simulink model "LoadFlow116BusNetwork_original"  (R2024a)
settings: Solver=FixedStepDiscrete  StartTime=0.0  StopTime=4.5  FixedStep=75e-6  RelTol=1e-3  EnableMultiTasking=on
undefined symbols (not defined in the file or in its folder): D1, D11, Delta
libraries: spsSeriesRLCBranchLib x164, spsLoadFlowBusLib x116, spsDistributedParametersLineLib x79, spsThreePhaseSeriesRLCLoadLib x60, spsThreePhaseTransformerTwoWindingsLib x52, spsThreePhaseParallelRLCLoadLib x44, spsThreePhaseVIMeasurementLib x44, spsSynchronousMachinepuStandardLib x28, spsExcitationSystemLib x28, spsHydraulicTurbineandGovernorLib x28, spsGenericPowerSystemStabilizerLib x28, spsMultiBandPowerSystemStabilizerLib x28
(part 9 of 15)

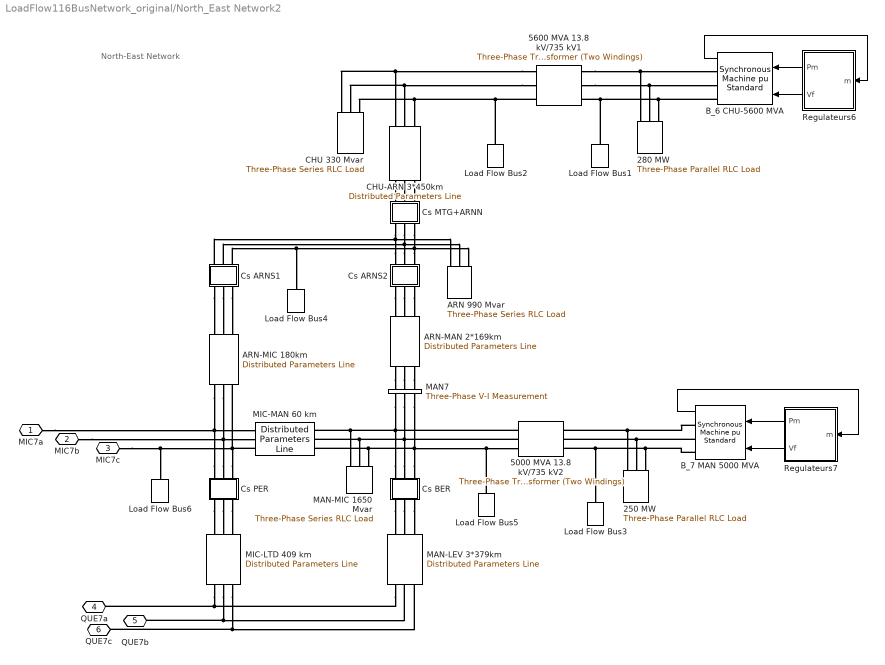
== system LoadFlow116BusNetwork_original/North_East Network2 ==
  note: North-East Network
  250 MW : spsThreePhaseParallelRLCLoadLib/Three-Phase Parallel RLC Load  LConnTagsString=A|B|C  Configuration=Y (grounded)  NominalVoltage=(13800)*1  Vabc=[1e3 1e3 1e3]  Vabcp=[1e3 1e3 1e3]  NominalFrequency=60  UnbalancedPower=off  ActivePower=250000000  InductivePower=0  CapacitivePower=0  Pabc=[10e3 9e3 11e3]  QLabc=[100 90 110]  QCabc=[100 90 110]  Pabcp=[10e3 9e3 11e3]  QLabcp=[100 90 110]  QCabcp=[100 90 110]  Measurements=None  LoadType=constant PQ
  280 MW : spsThreePhaseParallelRLCLoadLib/Three-Phase Parallel RLC Load  LConnTagsString=A|B|C  Configuration=Y (grounded)  NominalVoltage=(13800)*1  Vabc=[1e3 1e3 1e3]  Vabcp=[1e3 1e3 1e3]  NominalFrequency=60  UnbalancedPower=off  ActivePower=280000000  InductivePower=0  CapacitivePower=0  Pabc=[10e3 9e3 11e3]  QLabc=[100 90 110]  QCabc=[100 90 110]  Pabcp=[10e3 9e3 11e3]  QLabcp=[100 90 110]  QCabcp=[100 90 110]  Measurements=None  LoadType=constant PQ
  5000 MVA 13.8 kV/735 kV2 : spsThreePhaseTransformerTwoWindingsLib/Three-Phase Transformer (Two Windings)  Winding1Connection=Delta (D1)  Winding2Connection=Yg  CoreType=Three single-phase transformers  SetSaturation=off  Hysteresis=off  DataFile='basic_model'  SetInitialFlux=off  Measurements=None  UNITS=pu  NominalPower=[ 5000e6 60 ]  Winding1="[ 13.8e3 0.002  0.0]"  Winding2=[ 735e3 0.002 0.12]  Rm=500  Lm=500  L0=0.5  Saturation="[ 0,0  ;  0.005,1.2  ;  1.0,1.4 ]"  InitialFluxes=[ 0.8 , -0.8 , 0.7 ]  BreakLoop=off  DiscreteSolver=Trapezoidal iterative  DataType=off  TransfoNumber=0
  5600 MVA 13.8 kV/735 kV1 : spsThreePhaseTransformerTwoWindingsLib/Three-Phase Transformer (Two Windings)  Winding1Connection=Delta (D1)  Winding2Connection=Yg  CoreType=Three single-phase transformers  SetSaturation=off  Hysteresis=off  DataFile='basic_model'  SetInitialFlux=off  Measurements=None  UNITS=pu  NominalPower=[ 5600e6 60 ]  Winding1="[ 13.8e3 0.002  0.0]"  Winding2=[ 735e3 0.002 0.12]  Rm=500  Lm=500  L0=0.5  Saturation="[ 0,0  ;  0.005,1.2  ;  1.0,1.4 ]"  InitialFluxes=[ 0.8 , -0.8 , 0.7 ]  BreakLoop=off  DiscreteSolver=Trapezoidal iterative  DataType=off  TransfoNumber=0
  ARN 990 Mvar : spsThreePhaseSeriesRLCLoadLib/Three-Phase Series RLC Load  LConnTagsString=A|B|C  Configuration=Y (grounded)  NominalVoltage=735e3  Vabc=[1e3 1e3 1e3]  Vabcp=[1e3 1e3 1e3]  NominalFrequency=60  UnbalancedPower=off  ActivePower=3300000  InductivePower=990e6  CapacitivePower=0  Pabc=[10e3 9e3 11e3]  QLabc=[100 90 110]  QCabc=[100 90 110]  Pabcp=[10e3 9e3 11e3]  QLabcp=[100 90 110]  QCabcp=[100 90 110]  Measurements=None  LoadType=constant Z
  ARN-MAN 2*169km : spsDistributedParametersLineLib/Distributed Parameters Line  Phases=3  Length=169  Frequency=60  Resistance="[0.01273  0.3864]/2"  Inductance="[0.9337e-3  4.1264e-3]/2"  Capacitance=[12.74e-9 7.751e-9]*2  x1=[-0.000975 -2.39586870846483e-10 276427.296115276 -784420.047795566;-0.0009 -2.90591302561273e-10 298492.841238361 -776291.834335347;-0.000825 -3.41363440034991e-10 320319.775751254 -767543.065060424;-0.00075 -3.91862696797781e-10 341890.651536468 -758180.733603095;-0.000675 -4.42048704516452e-10 363188.225165946 -748212.324067877;-0.0006 -4.91881345264304e-10 384195.471685193 -737645.805048832;-0.000525 -5.41320783590788e-10 404895.598222762 -726489.62325959;-0.00045 -5.90327498365356e-10 425272.057414223 -714752.696781179;-0.000375 -6.38862314370044e-10 445308.560629867 -702444.407933044;-0.0003 -6.86886433615546e-10 464989.090995594 -689574.595772967;-0.000225 -7.3436146635573e-10 484297.91619655 -676153.548231873;-0.00015 -7.81249461775817e-10 503219.601053305 -662191.99388982;-7.5e-05 -8.27512938329678e-10 521739.019860496 -647701.093399729]  x2=[-0.000975 7.40195009315087e-10 170603.864508994 -782532.609847174;-0.0009 7.0387327325566e-10 192658.333571074 -777396.800423905;-0.000825 6.66988871671214e-10 214558.794509069 -771639.551892947;-0.00075 6.29571289388027e-10 236287.740429593 -765265.466510687;-0.000675 5.91650437448866e-10 257827.801545741 -758279.639623453;-0.0006 5.53256629202564e-10 279161.759062231 -750687.655594371;-0.000525 5.14420556071987e-10 300272.558939845 -742495.583339313;-0.00045 4.75173263019785e-10 321143.325528167 -733709.971475497;-0.000375 4.3554612373152e-10 341757.375055719 -724337.843086623;-0.0003 3.95570815536023e-10 362098.228966715 -714386.690108725;-0.000225 3.55279294083023e-10 382149.627093764 -703864.467341238;-0.00015 3.14703767798289e-10 401895.540655999 -692779.586088046;-7.5e-05 2.73876672136705e-10 421320.185072241 -681140.907433618]  x3=[-0.000975 -2.27971503827804e-12 1329.17201367258 -2414.87241463385;-0.0009 -2.23116849943949e-12 1396.90953145547 -2376.33167069258;-0.000825 -2.1808383986405e-12 1463.53038113235 -2335.89132357285;-0.00075 -2.12876496899359e-12 1528.98130701531 -2293.58370066939;-0.000675 -2.07498983720166e-12 1593.20998863565 -2249.44262204862;-0.0006 -2.01955599028229e-12 1656.165082568 -2203.50337341342;-0.000525 -1.96250774120452e-12 1717.79626347352 -2155.80267789624;-0.00045 -1.90389069346581e-12 1778.05426432918 -2106.37866670323;-0.000375 -1.84375170463725e-12 1836.89091581108 -2055.27084863274;-0.0003 -1.78213884890635e-12 1894.25918480026 -2002.52007849255;-0.000225 -1.71910137864727e-12 1950.11321198024 -1948.1685244412;-0.00015 -1.65468968504923e-12 2004.4083484963 -1892.25963427938;-7.5e-05 -1.58895525783457e-12 2057.10119164705 -1834.83810071847]  x4=[-0.000975 6.31095550685803e-12 681.724417843018 -9455.17189861404;-0.0009 5.98193937673865e-12 948.756484624173 -9432.1197918928;-0.000825 5.64814137580825e-12 1215.03012998798 -9401.5277929262;-0.00075 5.30982833708149e-12 1480.33249885646 -9363.42035649013;-0.000675 4.96727070282516e-12 1744.4515125752 -9317.82794508622;-0.0006 4.62074230837078e-12 2007.17603844579 -9264.78700459055;-0.000525 4.27052016321482e-12 2268.29605850207 -9204.33993511941;-0.00045 3.91688422958154e-12 2527.60283739528 -9136.53505713526;-0.000375 3.56011719862547e-12 2784.88908925389 -9061.4265728201;-0.0003 3.20050426445244e-12 3039.94914338479 -8979.07452274711;-0.000225 2.83833289613976e-12 3292.57910868325 -8889.54473788509;-0.00015 2.47389260793785e-12 3542.57703662037 -8792.9087869742;-7.5e-05 2.10747472783699e-12 3789.74308267767 -8689.24391931501]  x5=0.000955765248222805  V1=ones(3,3)  V2=ones(3,3)  I1=ones(3,3)  I2=ones(3,3)  nHarmo=1  Measurements=None  Decoupling=off  VsMag0=[ 1 1 1]  VrMag0=[ 1 1 1]  VsAngle0=[0 -120 120]  VrAngle0=[0 -120 120]  IsMag0=[ 1 1 1]  IrMag0=[ 1 1 1]  IsAngle0=[0 -120 120]  IrAngle0=[0 -120 120]
      settings: AttributesFormatString=\n  LibrarySourceBlock=sps_lib/Power Grid Elements/Distributed Parameters Line
  ARN-MIC 180km : spsDistributedParametersLineLib/Distributed Parameters Line  Phases=3  Length=180  Frequency=60  Resistance="[0.01273  0.3864]"  Inductance="[0.9337e-3  4.1264e-3]"  Capacitance=[12.74e-9 7.751e-9]  x1=[-0.00105 1.17005537388899e-10 262529.955827567 -774207.772445569;-0.000975 4.07599497187105e-11 284312.349574821 -766476.523484187;-0.0009 -3.55182208316351e-11 305867.468379951 -758132.564917417;-0.000825 -1.11767998659695e-10 327178.081410786 -749182.566778069;-0.00075 -1.87928430859734e-10 348227.153289335 -739633.683557717;-0.000675 -2.63938635947545e-10 368997.857709598 -729493.548487502;-0.0006 -3.39737852528176e-10 389473.590888265 -718770.267436253;-0.000525 -4.1526548786766e-10 409637.984837521 -707472.412430769;-0.00045 -4.90461166329917e-10 429474.92044937 -695609.014803479;-0.000375 -5.65264777640118e-10 448968.540380998 -683189.55797293;-0.0003 -6.39616524935914e-10 468103.261730894 -670223.969862888;-0.000225 -7.13456972568138e-10 486863.788495583 -656722.614966108;-0.00015 -7.86727093612748e-10 505235.123797014 -642696.286059117;-7.5e-05 -8.59368317056052e-10 523202.581870839 -628156.195574634]  x2=[-0.00105 9.8594506528747e-10 126759.491965791 -811882.989724261;-0.000975 9.6152968742284e-10 149661.239004331 -807974.954382946;-0.0009 9.36345677437981e-10 172443.349138306 -803421.03622553;-0.000825 9.10413167045148e-10 195087.610697451 -798224.875584509;-0.00075 8.83752886296367e-10 217575.922205545 -792390.626191196;-0.000675 8.56386147012154e-10 239890.306850452 -785922.951855288;-0.0006 8.28334825745166e-10 262012.926854506 -778827.022736693;-0.000525 7.99621346292426e-10 283926.097733766 -771108.511212574;-0.00045 7.70268661770077e-10 305612.302434712 -762773.587342948;-0.000375 7.40300236265014e-10 327054.205337117 -753828.913938427;-0.0003 7.09740026078054e-10 348234.666111872 -744281.641234073;-0.000225 6.78612460573634e-10 369136.753422707 -734139.401173607;-0.00015 6.46942422651351e-10 389743.758460837 -723410.301308553;-7.5e-05 6.1475522885495e-10 410039.208301734 -712102.918317182]  x3=[-0.00105 -6.27014655896914e-12 -44.8517351578419 -825.879343626748;-0.000975 -6.21302133868363e-12 -21.4861584031567 -826.817643960627;-0.0009 -6.15092952420239e-12 1.89659405780674 -827.094998920659;-0.000825 -6.08392075077187e-12 25.2778304104992 -826.71118679353;-0.00075 -6.0120485841803e-12 48.6388600523253 -825.666514392785;-0.000675 -5.93537047793796e-12 71.9610085336252 -823.961816813555;-0.0006 -5.85394772734977e-12 95.2256324857436 -821.598456765003;-0.000525 -5.76784542051675e-12 118.414134524254 -818.578323480991;-0.00045 -5.67713238630555e-12 141.507978115423 -814.903831209856;-0.000375 -5.58188113932778e-12 164.48870239403 -810.577917284499;-0.0003 -5.48216782197288e-12 187.337936920706 -805.604039774323;-0.000225 -5.37807214354107e-12 210.037416366974 -799.986174720907;-0.00015 -5.26967731652498e-12 232.568995116278 -793.728812959617;-7.5e-05 -5.15706999009083e-12 254.914661769311 -786.836956529706]  x4=[-0.00105 6.84257300336269e-12 787.856966726218 -5164.0243704381;-0.000975 6.69483696503938e-12 933.532622339274 -5139.68710729493;-0.0009 6.54174917648066e-12 1078.46202625756 -5111.24125691804;-0.000825 6.38343201372237e-12 1222.52932413308 -5078.70955848498;-0.00075 6.22001203308211e-12 1365.61935077221 -5042.11801733773;-0.000675 6.05161986999197e-12 1507.61772219701 -5001.49588419441;-0.0006 5.87839013457065e-12 1648.41092708201 -4956.87563176672;-0.000525 5.70046130401813e-12 1787.88641749343 -4908.29292880174;-0.00045 5.51797561191918e-12 1925.93269885829 -4855.78661156888;-0.000375 5.3310789345439e-12 2062.43941909144 -4799.39865281475;-0.0003 5.1399206742366e-12 2197.29745680935 -4739.17412821082;-0.000225 4.94465363998574e-12 2330.39900856007 -4675.1611803206;-0.00015 4.74543392527081e-12 2461.63767499964 -4607.4109801152;-7.5e-05 4.54242078328359e-12 2590.90854594614 -4535.97768606804]  x5=0.00101797482059234  V1=ones(3,3)  V2=ones(3,3)  I1=ones(3,3)  I2=ones(3,3)  nHarmo=1  Measurements=None  Decoupling=off  VsMag0=[ 1 1 1]  VrMag0=[ 1 1 1]  VsAngle0=[0 -120 120]  VrAngle0=[0 -120 120]  IsMag0=[ 1 1 1]  IrMag0=[ 1 1 1]  IsAngle0=[0 -120 120]  IrAngle0=[0 -120 120]
      settings: AttributesFormatString=\n  LibrarySourceBlock=sps_lib/Power Grid Elements/Distributed Parameters Line
  "B_6 CHU-5600 MVA " : spsSynchronousMachinepuStandardLib/Synchronous Machine pu Standard  PresetModel=No  MechanicalLoad=Mechanical power Pm  ShowDetailedParameters=on  RotorType=Salient-pole  Units=per unit standard parameters  MeasurementBus=off  NominalParameters="[ 5600E6  13800   60 ]"  Reactances1=[ 31 32 33 34 35 36 37 ]  Reactances2=[ 1.305, 0.296, 0.252, 0.474, 0.243, 0.18 ]  dAxisTimeConstants=Short-circuit  qAxisTimeConstants=Open-circuit  TimeConstants1=[]  TimeConstants2=[]  TimeConstants3=[]  TimeConstants4=[]  TimeConstants5=[ 1.01, 0.053, 0.1 ]  TimeConstants6=[]  TimeConstants7=[]  TimeConstants8=[]  StatorResistance=2.8544e-3  Mechanical="[ 4.0 0  32]"  PolePairs=32  InitialConditions=[0 -61.7964 0.894782 0.894782 0.894782 8.48442 -111.516 128.484 1.31361]  SetSaturation=off  Saturation=[0.6404,0.7127,0.8441,0.9214,0.9956,1.082,1.19,1.316,1.457;0.7,0.7698,0.8872,0.9466,0.9969,1.046,1.1,1.151,1.201]  LoadFlowParameters=[1 5000000000 0 0 0]  TsPowergui=0  TsBlock=-1  IterativeModel=Trapezoidal non iterative  IterativeDiscreteModel=Trapezoidal non iterative  BusType=PV  Pref=5000000000  Qref=0  Qmin=-Inf  Qmax=Inf  PLF=0  QLF=0
  B_7 MAN 5000 MVA : spsSynchronousMachinepuStandardLib/Synchronous Machine pu Standard  PresetModel=No  MechanicalLoad=Mechanical power Pm  ShowDetailedParameters=on  RotorType=Salient-pole  Units=per unit standard parameters  MeasurementBus=off  NominalParameters="[ 5000E6  13800   60 ]"  Reactances1=[ 31 32 33 34 35 36 37 ]  Reactances2=[ 1.305, 0.296, 0.252, 0.474, 0.243, 0.18 ]  dAxisTimeConstants=Short-circuit  qAxisTimeConstants=Open-circuit  TimeConstants1=[]  TimeConstants2=[]  TimeConstants3=[]  TimeConstants4=[]  TimeConstants5=[ 1.01, 0.053, 0.1 ]  TimeConstants6=[]  TimeConstants7=[]  TimeConstants8=[]  StatorResistance=2.8544e-3  Mechanical="[ 3.7 0  32]"  PolePairs=32  InitialConditions=[0 -81.9543 0.907703 0.907703 0.907703 -8.76021 -128.76 111.24 1.25655]  SetSaturation=off  Saturation=[0.6404,0.7127,0.8441,0.9214,0.9956,1.082,1.19,1.316,1.457;0.7,0.7698,0.8872,0.9466,0.9969,1.046,1.1,1.151,1.201]  LoadFlowParameters=[1 4500000000 0 0 0]  TsPowergui=0  TsBlock=-1  IterativeModel=Trapezoidal non iterative  IterativeDiscreteModel=Trapezoidal non iterative  BusType=PV  Pref=4500000000  Qref=0  Qmin=-Inf  Qmax=Inf  PLF=0  QLF=0
  CHU 330 Mvar : spsThreePhaseSeriesRLCLoadLib/Three-Phase Series RLC Load  LConnTagsString=A|B|C  Configuration=Y (grounded)  NominalVoltage=735e3  Vabc=[1e3 1e3 1e3]  Vabcp=[1e3 1e3 1e3]  NominalFrequency=60  UnbalancedPower=off  ActivePower=1100000  InductivePower=330e6  CapacitivePower=0  Pabc=[10e3 9e3 11e3]  QLabc=[100 90 110]  QCabc=[100 90 110]  Pabcp=[10e3 9e3 11e3]  QLabcp=[100 90 110]  QCabcp=[100 90 110]  Measurements=None  LoadType=constant Z
  CHU-ARN 3*450km : spsDistributedParametersLineLib/Distributed Parameters Line  Phases=3  Length=450  Frequency=60  Resistance="[0.01273  0.3864]/3"  Inductance="[0.9337e-3  4.1264e-3]/3"  Capacitance=[12.74e-9 7.751e-9]*3  x1=[-0.00255 1.7339566541592e-09 0 0;-0.002475 1.72011384974405e-09 0 0;-0.0024 1.70489601263604e-09 0 0;-0.002325 1.68831530774132e-09 0 0;-0.00225 1.67038498942168e-09 0 0;-0.002175 1.65111939089924e-09 0 0;-0.0021 1.63053391279869e-09 0 0;-0.002025 1.60864501083626e-09 0 0;-0.00195 1.58547018266525e-09 0 0;-0.001875 1.56102795388873e-09 0 0;-0.0018 1.53533786325041e-09 0 0;-0.001725 1.50842044701565e-09 0 0;-0.00165 1.48029722255516e-09 0 0;-0.001575 1.45099067114427e-09 242668.421457248 -732167.508894387;-0.0015 1.42052421999176e-09 263270.288908911 -725014.590467163;-0.001425 1.38892222351254e-09 283661.70211979 -717282.106469415;-0.00135 1.35620994385907e-09 303826.360506165 -708976.23813054;-0.001275 1.32241353072719e-09 323748.144748649 -700103.625034604;-0.0012 1.28756000045244e-09 343411.129677735 -690671.359812759;-0.001125 1.25167721441367e-09 362799.597004123 -680686.982473506;-0.00105 1.21479385676099e-09 381898.047883686 -670158.474375324;-0.000975 1.17693941148619e-09 400691.215307006 -659094.251846495;-0.0009 1.13814413885363e-09 419164.076303591 -647503.15945722;-0.000825 1.09843905121065e-09 437301.863951005 -635394.462949406;-0.00075 1.05785588819682e-09 455090.079179319 -622777.841829771;-0.000675 1.0164270913717e-09 472514.502361449 -609663.381632197;-0.0006 9.741857782816e-10 489561.204680105 -596061.56585551;-0.000525 9.31165715985879e-10 506216.559262278 -581983.267583126;-0.00045 8.87401294064112e-10 522467.252072349 -567439.740791278;-0.000375 8.42927497125565e-10 538300.292555131 -552442.61135276;-0.0003 7.9777987684304e-10 553703.024020315 -537003.867743383;-0.000225 7.51994523533407e-10 568663.133760038 -521135.851458566;-0.00015 7.05608037307564e-10 583168.66289147 -504851.24714774;-7.5e-05 6.58657498812863e-10 597208.015916567 -488163.072474426]  x2=[-0.00255 1.2084880276932e-09 0 0;-0.002475 1.16207776398563e-09 0 0;-0.0024 1.11473855309391e-09 0 0;-0.002325 1.06650823725891e-09 0 0;-0.00225 1.01742537105718e-09 0 0;-0.002175 9.67529190580951e-10 0 0;-0.0021 9.16859582073467e-10 0 0;-0.002025 8.65457050044495e-10 0 0;-0.00195 8.13362684891654e-10 0 0;-0.001875 7.60618130053377e-10 0 0;-0.0018 7.07265548719783e-10 0 0;-0.001725 6.53347590128069e-10 0 0;-0.00165 5.98907355469359e-10 0 0;-0.001575 5.43988363434277e-10 -54170.2857365492 -807523.190587187;-0.0015 4.88634515424766e-10 -31319.4766464824 -808731.868853793;-0.001425 4.32890060459984e-10 -8443.63124598836 -809294.05923845;-0.00135 3.76799559804311e-10 14438.9638641318 -809209.312334767;-0.001275 3.20407851345756e-10 37310.0166874625 -808477.69588812;-0.0012 2.6376001375324e-10 60151.2444543155 -807099.794741505;-0.001125 2.06901330441393e-10 82944.3882366968 -805076.710368013;-0.00105 1.49877253371688e-10 105671.227544213 -802410.059990341;-0.000975 9.27333667188362e-11 128313.594889255 -799101.975287998;-0.0009 3.55153504314977e-11 150853.390309806 -795155.100693279;-0.000825 -2.17310562835728e-11 173272.595838278 -790572.591277348;-0.00075 -7.89600915247464e-11 195553.289904796 -785358.110228115;-0.000675 -1.36126007276885e-10 217677.66166343 -779515.825921949;-0.0006 -1.93183105981604e-10 239628.02522991 -773050.408591532;-0.000525 -2.50085777067203e-10 261386.833819453 -765967.026592556;-0.00045 -3.06788533409054e-10 282936.693773393 -758271.342272209;-0.000375 -3.6324604769132e-10 304260.378463408 -749969.507442791;-0.0003 -4.19413188640913e-10 325340.842062219 -741068.158464041;-0.000225 -4.75245057104743e-10 346161.233169767 -731574.410938139;-0.00015 -5.30697021941417e-10 366704.908283963 -721495.854021596;-7.5e-05 -5.85724755698687e-10 386955.445105251 -710840.544358605]  x3=[-0.00255 1.12426609472525e-11 0 0;-0.002475 1.12250127765922e-11 0 0;-0.0024 1.11983915024668e-11 0 0;-0.002325 1.11628184055155e-11 0 0;-0.00225 1.11183219223276e-11 0 0;-0.002175 1.1064937622711e-11 0 0;-0.0021 1.10027081812581e-11 0 0;-0.002025 1.09316833432322e-11 0 0;-0.00195 1.0851919884802e-11 0 0;-0.001875 1.07634815676559e-11 0 0;-0.0018 1.06664390880314e-11 0 0;-0.001725 1.05608700202018e-11 0 0;-0.00165 1.04468587544649e-11 0 0;-0.001575 1.0324496429682e-11 -1464.09976004762 -2947.404391749;-0.0015 1.01938808604232e-11 -1380.19037065049 -2987.61903902351;-0.001425 1.00551164587763e-11 -1295.17767818868 -3025.44542935033;-0.00135 9.90831415088063e-12 -1209.1296405078 -3060.8533248918;-0.001275 9.75359128825505e-12 -1122.11504309261 -3093.81442111797;-0.0012 9.59107155398859e-12 -1034.20344408091 -3124.30236943285;-0.001125 9.42088486387018e-12 -945.465118659855 -3152.29279823704;-0.00105 9.24316726253597e-12 -855.971002889042 -3177.76333241001;-0.000975 9.05806081471729e-12 -765.792636995315 -3200.69361119647;-0.0009 8.8657134916763e-12 -675.002108184594 -3221.06530448238;-0.000825 8.66627905292003e-12 -583.67199301647 -3238.86212744785;-0.00075 8.45991692328738e-12 -491.875299387609 -3254.06985358489;-0.000675 8.24679206550732e-12 -399.685408170362 -3266.6763260699;-0.0006 8.02707484833023e-12 -307.176014553215 -3276.67146748169;-0.000525 7.80094091033776e-12 -214.421069129985 -3284.04728785712;-0.00045 7.56857101953997e-12 -121.494718784845 -3288.79789107825;-0.000375 7.33015092887217e-12 -28.4712474204399 -3290.91947958554;-0.0003 7.0858712277069e-12 64.5749834235285 -3290.41035741361;-0.000225 6.83592718949967e-12 157.569594013778 -3287.27093154693;-0.00015 6.58051861569035e-12 250.438245881469 -3281.50371159451;-7.5e-05 6.31984967598495e-12 343.106701247236 -3273.11330778372]  x4=[-0.00255 4.50201859654899e-12 0 0;-0.002475 4.38353361967566e-12 0 0;-0.0024 4.26154451309708e-12 0 0;-0.002325 4.13614879303855e-12 0 0;-0.00225 4.00744669892005e-12 0 0;-0.002175 3.87554111322643e-12 0 0;-0.0021 3.74053747926467e-12 0 0;-0.002025 3.60254371687413e-12 0 0;-0.00195 3.46167013615708e-12 0 0;-0.001875 3.31802934929852e-12 0 0;-0.0018 3.17173618054568e-12 0 0;-0.001725 3.0229075744193e-12 0 0;-0.00165 2.87166250222997e-12 0 0;-0.001575 2.71812186697426e-12 -1565.83540458769 -14460.8260986631;-0.0015 2.56240840668676e-12 -1156.3918700547 -14499.3124213113;-0.001425 2.40464659632511e-12 -746.02393355418 -14526.2082154568;-0.00135 2.24496254826669e-12 -335.059636935721 -14541.4919810133;-0.001275 2.08348391149626e-12 76.1725012299185 -14545.1515003725;-0.0012 1.92033976956536e-12 487.343748263553 -14537.1838481706;-0.001125 1.75566053740485e-12 898.125420161435 -14517.5953936267;-0.00105 1.58957785707324e-12 1308.18914434022 -14486.4017954519;-0.000975 1.42222449252405e-12 1717.20712213298 -14443.6279893312;-0.0009 1.2537342234763e-12 2124.85239082647 -14389.3081679908;-0.000825 1.08424173847307e-12 2530.79908503005 -14323.4857538646;-0.00075 9.1388252721357e-13 2934.72269716759 -14246.2133643835;-0.000675 7.42792772244684e-13 3336.30033688378 -14157.5527699132;-0.0006 5.71109240098776e-13 3735.21098915776 -14057.5748443766;-0.000525 3.98969171964597e-13 4131.13577091766 -13946.3595085974;-0.00045 2.26510173978783e-13 4523.75818595079 -13823.9956664135;-0.000375 5.38701072256124e-14 4912.76437790588 -13690.5811336081;-0.0003 -1.18813022467034e-13 5297.8433811851 -13546.2225597174;-0.000225 -2.91401174847421e-13 5678.68736952512 -13391.0353427767;-0.00015 -4.63756385587222e-13 6054.99190206876 -13225.1435370726;-7.5e-05 -6.35740876568096e-13 6426.45616673038 -13048.6797539765]  x5=0.00254493705148084  V1=ones(3,3)  V2=ones(3,3)  I1=ones(3,3)  I2=ones(3,3)  nHarmo=1  Measurements=None  Decoupling=off  VsMag0=[ 1 1 1]  VrMag0=[ 1 1 1]  VsAngle0=[0 -120 120]  VrAngle0=[0 -120 120]  IsMag0=[ 1 1 1]  IrMag0=[ 1 1 1]  IsAngle0=[0 -120 120]  IrAngle0=[0 -120 120]
      settings: AttributesFormatString=\n  LibrarySourceBlock=sps_lib/Power Grid Elements/Distributed Parameters Line
  "Cs ARNS1 " : Subsystem  mask{Xc=25}
      mask prompts: Xc "Condensator Reactance at  60Hz  (ohm):"
      mask help: Series Compensation
      mask init:
      | Cs=1/Xc/(2*pi*60);
      mask Display: disp('Cs')
  Cs ARNS2 : Subsystem  mask{Xc=25/2}
      mask prompts: Xc "Condensator Reactance at  60Hz  (ohm):"
      mask help: Series Compensation
      mask init:
      | Cs=1/Xc/(2*pi*60);
      mask Display: disp('Cs')
  Cs BER : Subsystem  mask{Xc=22/3}
      mask prompts: Xc "Condensator Reactance at  60Hz  (ohm):"
      mask help: Series Compensation
      mask init:
      | Cs=1/Xc/(2*pi*60);
      mask Display: disp('Cs')
  "Cs MTG+ARNN " : Subsystem  mask{Xc=(30+25)/3}
      mask prompts: Xc "Condensator Reactance at  60Hz  (ohm):"
      mask help: Series Compensation
      mask init:
      | Cs=1/Xc/(2*pi*60);
      mask Display: disp('Cs')
  "Cs PER " : Subsystem  mask{Xc=22}
      mask prompts: Xc "Condensator Reactance at  60Hz  (ohm):"
      mask help: Series Compensation
      mask init:
      | Cs=1/Xc/(2*pi*60);
      mask Display: disp('Cs')
  Load Flow Bus1 : spsLoadFlowBusLib/Load Flow Bus  LConnTagsString=a  Phases=single  Connectors=on one side  ID=CHU_13.8  Vbase=13.8e3  Vref=1  Vangle=0  VLF=1  VLFb=1  VLFc=1  angleLF=4.726  angleLFb=0  angleLFc=0
      settings: AttributesFormatString=%<ID>\n%<Vbase>V\n%<VLF>pu\n%<angleLF>deg.
  Load Flow Bus2 : spsLoadFlowBusLib/Load Flow Bus  LConnTagsString=a  Phases=single  Connectors=on one side  ID=CHU7  Vbase=735e3  Vref=1  Vangle=0  VLF=1.009  VLFb=1  VLFc=1  angleLF=28.97  angleLFb=0  angleLFc=0
      settings: AttributesFormatString=%<ID>\n%<Vbase>V\n%<VLF>pu\n%<angleLF>deg.
  Load Flow Bus3 : spsLoadFlowBusLib/Load Flow Bus  LConnTagsString=a  Phases=single  Connectors=on one side  ID=MAN_13.8  Vbase=13.8e3  Vref=1  Vangle=0  VLF=1  VLFb=1  VLFc=1  angleLF=-16.23  angleLFb=0  angleLFc=0
      settings: AttributesFormatString=%<ID>\n%<Vbase>V\n%<VLF>pu\n%<angleLF>deg.
  Load Flow Bus4 : spsLoadFlowBusLib/Load Flow Bus  LConnTagsString=a  Phases=single  Connectors=on one side  ID=ARN7  Vbase=735e3  Vref=1  Vangle=0  VLF=1.054  VLFb=1  VLFc=1  angleLF=12.72  angleLFb=0  angleLFc=0
      settings: AttributesFormatString=%<ID>\n%<Vbase>V\n%<VLF>pu\n%<angleLF>deg.
  Load Flow Bus5 : spsLoadFlowBusLib/Load Flow Bus  LConnTagsString=a  Phases=single  Connectors=on one side  ID=MAN7  Vbase=735e3  Vref=1  Vangle=0  VLF=1.016  VLFb=1  VLFc=1  angleLF=7.996  angleLFb=0  angleLFc=0
      settings: AttributesFormatString=%<ID>\n%<Vbase>V\n%<VLF>pu\n%<angleLF>deg.
  Load Flow Bus6 : spsLoadFlowBusLib/Load Flow Bus  LConnTagsString=a  Phases=single  Connectors=on one side  ID=MIC7  Vbase=735e3  Vref=1  Vangle=0  VLF=1.041  VLFb=1  VLFc=1  angleLF=5.981  angleLFb=0  angleLFc=0
      settings: AttributesFormatString=%<ID>\n%<Vbase>V\n%<VLF>pu\n%<angleLF>deg.
  MAN-LEV 3*379km : spsDistributedParametersLineLib/Distributed Parameters Line  Phases=3  Length=379  Frequency=60  Resistance="[0.01273  0.3864]/3"  Inductance="[0.9337e-3  4.1264e-3]/3"  Capacitance=[12.74e-9 7.751e-9]*3  x1=[-0.002175 3.40009767769328e-09 -129715.856575875 -778750.814672904;-0.0021 3.3630582454327e-09 -107648.25126904 -782106.718665414;-0.002025 3.32333043586723e-09 -85494.5935972146 -784837.418513656;-0.00195 3.2809460068e-09 -63272.5928553784 -786940.731337954;-0.001875 3.23593883969508e-09 -41000.0129709167 -788414.975782217;-0.0018 3.18834491259324e-09 -18694.6583034074 -789258.973357993;-0.001725 3.13820227135159e-09 3625.64058791194 -789472.049386535;-0.00165 3.08555099923032e-09 25943.0411976193 -789054.033538124;-0.001575 3.03043318485078e-09 48239.7033371353 -788005.259968234;-0.0015 2.97289288855045e-09 70497.8033958956 -786326.567050411;-0.001425 2.91297610716181e-09 92699.548589274 -784019.296706087;-0.00135 2.85073073724312e-09 114827.191181861 -781085.293331874;-0.001275 2.78620653679073e-09 136863.042674732 -777526.902325177;-0.0012 2.71945508546321e-09 158789.487945363 -773346.968209322;-0.001125 2.65052974334944e-09 180588.999328892 -768548.832359686;-0.00105 2.57948560831329e-09 202244.150629461 -763136.330332653;-0.000975 2.50637947194932e-09 223737.631050457 -757113.788799529;-0.0009 2.43126977418436e-09 245052.259032491 -750486.022087869;-0.000825 2.35421655656159e-09 266170.99598808 -743258.328332972;-0.00075 2.27528141424423e-09 287076.959922029 -735436.485242641;-0.000675 2.19452744677729e-09 307753.438926641 -727026.745478561;-0.0006 2.11201920764679e-09 328183.90454096 -718035.831658029;-0.000525 2.02782265267669e-09 348352.024963372 -708470.930979985;-0.00045 1.94200508730475e-09 368241.678106993 -698339.689479685;-0.000375 1.8546351127797e-09 387836.964487421 -687650.205916571;-0.0003 1.76578257132237e-09 407122.219932543 -676411.025300247;-0.000225 1.67551849029489e-09 426082.02810423 -664631.132059735;-0.00015 1.58391502542257e-09 444701.232821924 -652319.942861451;-7.5e-05 1.49104540311364e-09 462964.950178257 -639487.299081673]  x2=[-0.002175 1.76936071610415e-09 -453830.168531879 -672756.853007292;-0.0021 1.81200596388042e-09 -434629.546159923 -685317.991887154;-0.002025 1.85320272181379e-09 -415081.487578821 -697331.298050017;-0.00195 1.89291805784629e-09 -395201.619207509 -708787.168242747;-0.001875 1.93112022414597e-09 -375005.832708591 -719676.44481799;-0.0018 1.9677786824856e-09 -354510.272284786 -729990.423054665;-0.001725 2.00286412865447e-09 -333731.321773506 -739720.858116378;-0.00165 2.03634851588374e-09 -312685.591549861 -748859.971642221;-0.001575 2.06820507726659e-09 -291389.905248581 -757400.457964676;-0.0015 2.09840834715528e-09 -269861.28631546 -765335.489949649;-0.001425 2.12693418151797e-09 -248116.944399075 -772658.724453982;-0.00135 2.15375977723914e-09 -226174.261593654 -779364.307396061;-0.001275 2.17886369034802e-09 -204050.778544097 -785446.878435482;-0.0012 2.20222585316057e-09 -181764.180424253 -790901.575258022;-0.001125 2.22382759032128e-09 -159332.282799664 -795724.0374625;-0.00105 2.24365163373199e-09 -136773.01738607 -799910.410046417;-0.000975 2.26168213635572e-09 -114104.417715075 -803457.346487582;-0.0009 2.27790468488455e-09 -91344.6047184146 -806362.011419275;-0.000825 2.29230631126139e-09 -68511.7722423618 -808622.082896792;-0.00075 2.30487550304646e-09 -45624.1725038437 -810235.754253574;-0.000675 2.31560221262018e-09 -22700.1014998993 -811201.735545428;-0.0006 2.32447786521504e-09 242.115617860982 -811519.25458169;-0.000525 2.33149536577014e-09 23184.1391921008 -811188.0575425;-0.00045 2.33664910460293e-09 46107.6297201997 -810208.409181705;-0.000375 2.33993496189342e-09 68994.2625145706 -808581.092615214;-0.0003 2.34135031097759e-09 91825.742351135 -806307.408694992;-0.000225 2.34089402044701e-09 114583.818094245 -803389.174969176;-0.00015 2.33856645505338e-09 137250.297286361 -799828.724229156;-7.5e-05 2.33436947541683e-09 159807.060690827 -795628.902644778]  x3=[-0.002175 -1.95883916998323e-12 -1369.21748803889 -554.792265212858;-0.0021 -2.14095939977132e-12 -1352.98611909914 -593.27968063411;-0.002025 -2.32136817937302e-12 -1335.67319375716 -631.292837356146;-0.00195 -2.49992129277026e-12 -1317.29255170057 -668.801348243105;-0.001875 -2.67647600733613e-12 -1297.85888613341 -705.775229565282;-0.0018 -2.85089118793319e-12 -1277.38773203058 -742.184924967667;-0.001725 -3.02302740973471e-12 -1255.89545371945 -778.001329096844;-0.00165 -3.19274706967877e-12 -1233.39923179847 -813.19581086736;-0.001575 -3.35991449646599e-12 -1209.91704940322 -847.740236348981;-0.0015 -3.52439605901315e-12 -1185.46767783104 -881.606991256526;-0.001425 -3.68606027327581e-12 -1160.07066153546 -914.7690030243;-0.00135 -3.84477790735462e-12 -1133.74630250272 -947.199762447491;-0.001275 -4.00042208480137e-12 -1106.51564402267 -978.873344873224;-0.0012 -4.15286838604204e-12 -1078.40045386703 -1009.76443092433;-0.001125 -4.30199494783592e-12 -1049.42320688866 -1039.84832673927;-0.00105 -4.44768256069123e-12 -1019.60706705542 -1069.10098371203;-0.000975 -4.58981476415935e-12 -988.97586893328 -1097.4990177162;-0.0009 -4.72827793993153e-12 -957.554098633355 -1125.0197277979;-0.000825 -4.8629614026636e-12 -925.366874238051 -1151.64111432259;-0.00075 -4.99375748845618e-12 -892.43992572207 -1177.34189656118;-0.000675 -5.12056164091955e-12 -858.799574384255 -1202.1015297016;-0.0006 -5.24327249475438e-12 -824.472711806751 -1225.90022127194;-0.000525 -5.36179195678167e-12 -789.486778358285 -1248.71894696231;-0.00045 -5.47602528435687e-12 -753.869741258752 -1270.53946583251;-0.000375 -5.58588116110576e-12 -717.65007222265 -1291.34433489363;-0.0003 -5.69127176992131e-12 -680.856724699228 -1311.11692305167;-0.000225 -5.79211286316335e-12 -643.519110727539 -1329.84142440218;-0.00015 -5.88832383000489e-12 -605.667077424906 -1347.50287086528;-7.5e-05 -5.97982776087109e-12 -567.330883127598 -1364.08714415089]  x4=[-0.002175 1.98835221259479e-11 -9019.35016940806 -13700.3757737256;-0.0021 2.02734388906559e-11 -8628.42708034488 -13949.8814959023;-0.002025 2.06471493785086e-11 -8230.60655869302 -14188.2358962515;-0.00195 2.10043548510602e-11 -7826.20661609065 -14415.2484379126;-0.001875 2.13447697637212e-11 -7415.55052366436 -14630.7376505331;-0.0018 2.16681219940191e-11 -6998.96655361117 -14834.5312753336;-0.001725 2.19741530591283e-11 -6576.78771678281 -15026.4664028085;-0.00165 2.22626183224979e-11 -6149.35149648188 -15206.3896029536;-0.001575 2.25332871894099e-11 -5716.99957868289 -15374.1570479157;-0.0015 2.27859432913136e-11 -5280.07757889373 -15529.6346269662;-0.001425 2.30203846587868e-11 -4838.9347658759 -15672.6980537073;-0.00135 2.32364238829875e-11 -4393.92378244441 -15803.2329654245;-0.001275 2.34338882654654e-11 -3945.40036357053 -15921.1350145068;-0.0012 2.36126199562143e-11 -3493.72305201265 -16026.30995186;-0.001125 2.37724760798554e-11 -3039.25291170276 -16118.6737022484;-0.00105 2.39133288498494e-11 -2582.35323911737 -16198.1524315033;-0.000975 2.4035065670647e-11 -2123.38927286397 -16264.6826055444;-0.0009 2.41375892276964e-11 -1662.72790171478 -16318.2110411687;-0.000825 2.42208175652346e-11 -1200.73737132155 -16358.6949485637;-0.00075 2.42846841518021e-11 -737.786989845592 -16386.1019655132;-0.000675 2.43291379334268e-11 -274.246832738464 -16400.4101832672;-0.0006 2.43541433744358e-11 189.512553090636 -16401.6081640555;-0.000525 2.43596804858621e-11 653.120445484435 -16389.6949502304;-0.00045 2.43457448414237e-11 1116.20624338719 -16364.6800650328;-0.000375 2.43123475810614e-11 1578.39976309751 -16326.5835049792;-0.0003 2.42595154020343e-11 2039.33153418754 -16275.4357238769;-0.000225 2.41872905375777e-11 2498.63309485196 -16211.2776084794;-0.00015 2.40957307231434e-11 2955.93728645072 -16134.1604458026;-7.5e-05 2.3984909150246e-11 3410.87854701005 -16044.1458821263]  x5=0.00214340253891386  V1=ones(3,3)  V2=ones(3,3)  I1=ones(3,3)  I2=ones(3,3)  nHarmo=1  Measurements=None  Decoupling=off  VsMag0=[ 1 1 1]  VrMag0=[ 1 1 1]  VsAngle0=[0 -120 120]  VrAngle0=[0 -120 120]  IsMag0=[ 1 1 1]  IrMag0=[ 1 1 1]  IsAngle0=[0 -120 120]  IrAngle0=[0 -120 120]
      settings: AttributesFormatString=\n  LibrarySourceBlock=sps_lib/Power Grid Elements/Distributed Parameters Line
  MAN-MIC 1650 Mvar : spsThreePhaseSeriesRLCLoadLib/Three-Phase Series RLC Load  LConnTagsString=A|B|C  Configuration=Y (grounded)  NominalVoltage=735e3  Vabc=[1e3 1e3 1e3]  Vabcp=[1e3 1e3 1e3]  NominalFrequency=60  UnbalancedPower=off  ActivePower=5500000  InductivePower=1650e6  CapacitivePower=0  Pabc=[10e3 9e3 11e3]  QLabc=[100 90 110]  QCabc=[100 90 110]  Pabcp=[10e3 9e3 11e3]  QLabcp=[100 90 110]  QCabcp=[100 90 110]  Measurements=None  LoadType=constant Z
  MAN7 : spsThreePhaseVIMeasurementLib/Three-Phase V-I Measurement  VoltageMeasurement=no  SetLabelV=on  LabelV=Vabc_MAN7  Vpu=on  VpuLL=off  CurrentMeasurement=no  SetLabelI=on  LabelI=Iabc_MAN7  Ipu=on  Pbase=100e6  Vbase=735e3  OutputType=Magnitude  PhasorSimulation=off  PSBequivalent=0
  MIC-LTD 409 km : spsDistributedParametersLineLib/Distributed Parameters Line  Phases=3  Length=409  Frequency=60  Resistance="[0.01273  0.3864]"  Inductance="[0.9337e-3  4.1264e-3]"  Capacitance=[12.74e-9 7.751e-9]  x1=[-0.002325 1.13289758925303e-09 0 0;-0.00225 1.12719175155242e-09 0 0;-0.002175 1.12058485401222e-09 0 0;-0.0021 1.11308217808525e-09 0 0;-0.002025 1.10468972129584e-09 0 0;-0.00195 1.09541419244555e-09 0 0;-0.001875 1.08526300625022e-09 0 0;-0.0018 1.07424427741278e-09 0 0;-0.001725 1.06236681413646e-09 0 0;-0.00165 1.04964011108367e-09 0 0;-0.001575 1.03607434178612e-09 0 0;-0.0015 1.02168035051221e-09 0 0;-0.001425 1.00646964359834e-09 59193.0163104635 -807702.943453841;-0.00135 9.90454380250877e-10 82003.602334413 -805706.722469032;-0.001275 9.736473628263e-10 104748.635933354 -803066.431858008;-0.0012 9.56062026597185e-10 127409.935075437 -799784.182228684;-0.001125 9.37712429012248e-10 149969.384664858 -795862.597361196;-0.00105 9.18613238459039e-10 172408.951022787 -791304.812110483;-0.000975 8.9877972253826e-10 194710.696303214 -786114.469900339;-0.0009 8.78227735859075e-10 216856.792832189 -780295.719810911;-0.000825 8.56973707365179e-10 238829.537358994 -773853.213261991;-0.00075 8.35034627201753e-10 260611.36520785 -766792.10029474;-0.000675 8.124280331338e-10 282184.864318845 -759118.025454827;-0.0006 7.89171996526726e-10 303532.789166878 -750837.12328026;-0.000525 7.65285107900364e-10 324638.074547457 -741956.013397536;-0.00045 7.40786462068002e-10 345483.849218373 -732481.79523001;-0.000375 7.15695642872276e-10 366053.449386304 -722422.042322724;-0.0003 6.90032707530148e-10 386330.4320276 -711784.796288233;-0.000225 6.63818170599475e-10 406298.588032588 -700578.560378263;-0.00015 6.37072987579983e-10 425941.955162879 -688812.292686337;-7.5e-05 6.09818538161764e-10 445244.830811344 -676495.398986819]  x2=[-0.002325 1.67986224150682e-09 0 0;-0.00225 1.72530106844355e-09 0 0;-0.002175 1.76936071610415e-09 0 0;-0.0021 1.81200596388042e-09 0 0;-0.002025 1.85320272181379e-09 0 0;-0.00195 1.89291805784629e-09 0 0;-0.001875 1.93112022414597e-09 0 0;-0.0018 1.9677786824856e-09 0 0;-0.001725 2.00286412865447e-09 0 0;-0.00165 2.03634851588374e-09 0 0;-0.001575 2.06820507726659e-09 0 0;-0.0015 2.09840834715528e-09 0 0;-0.001425 2.12693418151797e-09 -248116.944399075 -772658.724453982;-0.00135 2.15375977723914e-09 -226174.261593654 -779364.307396061;-0.001275 2.17886369034802e-09 -204050.778544097 -785446.878435482;-0.0012 2.20222585316057e-09 -181764.180424253 -790901.575258022;-0.001125 2.22382759032128e-09 -159332.282799664 -795724.0374625;-0.00105 2.24365163373199e-09 -136773.01738607 -799910.410046417;-0.000975 2.26168213635572e-09 -114104.417715075 -803457.346487582;-0.0009 2.27790468488455e-09 -91344.6047184146 -806362.011419275;-0.000825 2.29230631126139e-09 -68511.7722423618 -808622.082896792;-0.00075 2.30487550304646e-09 -45624.1725038437 -810235.754253574;-0.000675 2.31560221262018e-09 -22700.1014998993 -811201.735545428;-0.0006 2.32447786521504e-09 242.115617860982 -811519.25458169;-0.000525 2.33149536577014e-09 23184.1391921008 -811188.0575425;-0.00045 2.33664910460293e-09 46107.6297201997 -810208.409181705;-0.000375 2.33993496189342e-09 68994.2625145706 -808581.092615214;-0.0003 2.34135031097759e-09 91825.742351135 -806307.408694992;-0.000225 2.34089402044701e-09 114583.818094245 -803389.174969176;-0.00015 2.33856645505338e-09 137250.297286361 -799828.724229156;-7.5e-05 2.33436947541683e-09 159807.060690827 -795628.902644778]  x3=[-0.002325 -1.55518349783134e-12 0 0;-0.00225 -1.49356581414343e-12 0 0;-0.002175 -1.43075419679601e-12 0 0;-0.0021 -1.36679885643495e-12 0 0;-0.002025 -1.30175091798078e-12 0 0;-0.00195 -1.23566237976023e-12 0 0;-0.001875 -1.16858607193957e-12 0 0;-0.0018 -1.10057561429297e-12 0 0;-0.001725 -1.03168537333967e-12 0 0;-0.00165 -9.6197041888424e-13 0 0;-0.001575 -8.91486479994596e-13 0 0;-0.0015 -8.20289900453045e-13 0 0;-0.001425 -7.48437593715927e-13 -412.085781583752 -775.7108295152;-0.00135 -6.75986997417873e-13 -389.991383898849 -787.050857738442;-0.001275 -6.0299602745703e-13 -367.585233068726 -797.76172954829;-0.0012 -5.29523031697987e-13 -344.885240227529 -807.834882837701;-0.001125 -4.55626743329379e-13 -321.909551402217 -817.26226528206;-0.00105 -3.81366233913476e-13 -298.676533006894 -826.036340776084;-0.000975 -3.06800866165282e-13 -275.20475716099 -834.150095458071;-0.0009 -2.31990246498886e-13 -251.512986842986 -841.597043316674;-0.000825 -1.56994177379008e-13 -227.620160891577 -848.371231375716;-0.00075 -8.18726095158251e-14 -203.545378866257 -854.467244452912;-0.000675 -6.68559394128817e-15 -179.307885779419 -859.880209488679;-0.0006 6.85067659947523e-14 -154.927056712192 -864.605799441589;-0.000525 1.43644362670245e-13 -130.422381326293 -868.640236747338;-0.00045 2.18667132240052e-13 -105.813448284291 -871.980296338472;-0.000375 2.93515102650066e-13 -81.119929590731 -874.62330822246;-0.0003 3.68128441577952e-13 -56.3615648666323 -876.56715961604;-0.000225 4.42447504262196e-13 -31.5581455699402 -877.810296634149;-0.00015 5.16412881181205e-13 -6.72949917453518 -878.351725532078;-7.5e-05 5.89965445544381e-13 18.1045266795451 -878.191013499848]  x4=[-0.002325 3.22529002643264e-12 0 0;-0.00225 3.26816490939e-12 0 0;-0.002175 3.30842727132339e-12 0 0;-0.0021 3.34604492711673e-12 0 0;-0.002025 3.38098780579153e-12 0 0;-0.00195 3.41322797454522e-12 0 0;-0.001875 3.44273966108021e-12 0 0;-0.0018 3.46949927420581e-12 0 0;-0.001725 3.49348542269673e-12 0 0;-0.00165 3.51467893239286e-12 0 0;-0.001575 3.53306286152684e-12 0 0;-0.0015 3.54862251426698e-12 0 0;-0.001425 3.56134545246496e-12 -1850.18013712839 -4788.09574636232;-0.00135 3.57122150559865e-12 -1714.07818949413 -4838.4875331247;-0.001275 3.57824277890229e-12 -1576.60603398147 -4885.01150698444;-0.0012 3.58240365967743e-12 -1437.87356372813 -4927.63047738869;-0.001125 3.58370082177963e-12 -1297.99167934814 -4966.31037538458;-0.00105 3.58213322827737e-12 -1157.07220027962 -5001.02028085349;-0.000975 3.57770213228089e-12 -1015.227775398 -5031.73244722806;-0.0009 3.57041107594055e-12 -872.571792966227 -5058.4223236724;-0.000825 3.56026588761522e-12 -729.218289993955 -5081.06857470766;-0.00075 3.54727467721323e-12 -585.281861078077 -5099.65309726725;-0.000675 3.5314478297094e-12 -440.877566797564 -5114.1610351682;-0.0006 3.51279799684346e-12 -296.120841735808 -5124.58079098692;-0.000525 3.49134008700645e-12 -151.127402203968 -5130.90403533004;-0.00045 3.46709125332319e-12 -6.01315373913303 -5133.12571349278;-0.000375 3.4400708799403e-12 139.105901548797 -5131.24404949961;-0.0003 3.41030056653083e-12 284.11375770742 -5125.26054752394;-0.000225 3.37780411102782e-12 428.894497675218 -5115.17999068569;-0.00015 3.3426074906006e-12 573.33238594388 -5101.01043722777;-7.5e-05 3.30473884088899e-12 717.311961075499 -5082.76321407441]  x5=0.00231306500901259  V1=ones(3,3)  V2=ones(3,3)  I1=ones(3,3)  I2=ones(3,3)  nHarmo=1  Measurements=None  Decoupling=off  VsMag0=[ 1 1 1]  VrMag0=[ 1 1 1]  VsAngle0=[0 -120 120]  VrAngle0=[0 -120 120]  IsMag0=[ 1 1 1]  IrMag0=[ 1 1 1]  IsAngle0=[0 -120 120]  IrAngle0=[0 -120 120]
      settings: AttributesFormatString=\n  LibrarySourceBlock=sps_lib/Power Grid Elements/Distributed Parameters Line
  MIC-MAN 60 km : spsDistributedParametersLineLib/Distributed Parameters Line  Phases=3  Length=60  Frequency=60  Resistance="[0.01273  0.3864]"  Inductance="[0.9337e-3  4.1264e-3]"  Capacitance=[12.74e-9 7.751e-9]  x1=[-0.000375 7.40300236265014e-10 327054.205337117 -753828.913938427;-0.0003 7.09740026078054e-10 348234.666111872 -744281.641234073;-0.000225 6.78612460573634e-10 369136.753422707 -734139.401173607;-0.00015 6.46942422651351e-10 389743.758460837 -723410.301308553;-7.5e-05 6.1475522885495e-10 410039.208301734 -712102.918317182]  x2=[-0.000375 4.3554612373152e-10 341757.375055719 -724337.843086623;-0.0003 3.95570815536023e-10 362098.228966715 -714386.690108725;-0.000225 3.55279294083023e-10 382149.627093764 -703864.467341238;-0.00015 3.14703767798289e-10 401895.540655999 -692779.586088046;-7.5e-05 2.73876672136705e-10 421320.185072241 -681140.907433618]  x3=[-0.000375 5.63269476007816e-12 2516.12263919193 -3470.38246360578;-0.0003 5.58920237955469e-12 2613.22665570735 -3397.86332962469;-0.000225 5.54124207616666e-12 2708.24169881791 -3322.62799568694;-0.00015 5.4888521886468e-12 2801.09181495191 -3244.73660376736;-7.5e-05 5.43207459666959e-12 2891.70278114719 -3164.25141905286]  x4=[-0.000375 7.27997733660617e-13 -263.637973265085 -2074.49907539878;-0.0003 7.85154099462121e-13 -204.885257541821 -2081.12319463909;-0.000225 8.41682825089776e-13 -145.968759678528 -2086.08369583986;-0.00015 8.97538722345233e-13 -86.9355766221447 -2089.37661365233;-7.5e-05 9.5267714087885e-13 -27.8328985959686 -2090.99931576838]  x5=0.000339324940197445  V1=ones(3,3)  V2=ones(3,3)  I1=ones(3,3)  I2=ones(3,3)  nHarmo=1  Measurements=None  Decoupling=off  VsMag0=[ 1 1 1]  VrMag0=[ 1 1 1]  VsAngle0=[0 -120 120]  VrAngle0=[0 -120 120]  IsMag0=[ 1 1 1]  IrMag0=[ 1 1 1]  IsAngle0=[0 -120 120]  IrAngle0=[0 -120 120]
      settings: AttributesFormatString=\n  LibrarySourceBlock=sps_lib/Power Grid Elements/Distributed Parameters Line
  Regulateurs6 : Subsystem
  Regulateurs7 : Subsystem
  "MIC7a " : PMIOPort  Side=Left
  MIC7b : PMIOPort  Port=2  Side=Left
  MIC7c : PMIOPort  Port=3  Side=Left
  QUE7a : PMIOPort  Port=4  Side=Left
  QUE7b : PMIOPort  Port=5  Side=Left
  QUE7c : PMIOPort  Port=6  Side=Left
  wires:
  Regulateurs6/1(Pm) -> "B_6 CHU-5600 MVA "/1
  Regulateurs6/2(Vf) -> "B_6 CHU-5600 MVA "/2
  "B_6 CHU-5600 MVA "/1 -> Regulateurs6/1(m)
  Regulateurs7/1(Pm) -> B_7 MAN 5000 MVA/1
  Regulateurs7/2(Vf) -> B_7 MAN 5000 MVA/2
  B_7 MAN 5000 MVA/1 -> Regulateurs7/1(m)
  connections:
  "Cs PER "/RConn3 -- MIC-LTD 409 km/LConn3
  "Cs PER "/RConn2 -- MIC-LTD 409 km/LConn2
  "Cs PER "/RConn1 -- MIC-LTD 409 km/LConn1
  Cs BER/RConn3 -- MAN-LEV 3*379km/LConn3
  Cs BER/RConn2 -- MAN-LEV 3*379km/LConn2
  Cs BER/RConn1 -- MAN-LEV 3*379km/LConn1
  Cs ARNS2/RConn3 -- ARN-MAN 2*169km/LConn3
  Cs ARNS2/RConn2 -- ARN-MAN 2*169km/LConn2
  Cs ARNS2/RConn1 -- ARN-MAN 2*169km/LConn1
  CHU-ARN 3*450km/RConn3 -- "Cs MTG+ARNN "/LConn3
  CHU-ARN 3*450km/RConn2 -- "Cs MTG+ARNN "/LConn2
  CHU-ARN 3*450km/RConn1 -- "Cs MTG+ARNN "/LConn1
  Load Flow Bus2/LConn1 -- 5600 MVA 13.8 kV/735 kV1/RConn3 -- CHU-ARN 3*450km/LConn3 -- CHU 330 Mvar/LConn3
  5600 MVA 13.8 kV/735 kV1/RConn2 -- CHU-ARN 3*450km/LConn2 -- CHU 330 Mvar/LConn2
  5600 MVA 13.8 kV/735 kV1/RConn1 -- CHU-ARN 3*450km/LConn1 -- CHU 330 Mvar/LConn1
  "B_6 CHU-5600 MVA "/RConn3 -- Load Flow Bus1/LConn1 -- 5600 MVA 13.8 kV/735 kV1/LConn3 -- 280 MW/LConn3
  5600 MVA 13.8 kV/735 kV1/LConn2 -- "B_6 CHU-5600 MVA "/RConn2 -- 280 MW/LConn2
  5600 MVA 13.8 kV/735 kV1/LConn1 -- "B_6 CHU-5600 MVA "/RConn1 -- 280 MW/LConn1
  "Cs ARNS1 "/RConn1 -- ARN-MIC 180km/LConn1
  "Cs ARNS1 "/RConn2 -- ARN-MIC 180km/LConn2
  "Cs ARNS1 "/RConn3 -- ARN-MIC 180km/LConn3
  "Cs PER "/LConn3 -- Load Flow Bus6/LConn1 -- MIC7c/RConn1 -- MIC-MAN 60 km/LConn3 -- ARN-MIC 180km/RConn3
  "Cs PER "/LConn2 -- MIC7b/RConn1 -- ARN-MIC 180km/RConn2 -- MIC-MAN 60 km/LConn2
  "Cs PER "/LConn1 -- "MIC7a "/RConn1 -- ARN-MIC 180km/RConn1 -- MIC-MAN 60 km/LConn1
  ARN-MAN 2*169km/RConn1 -- MAN7/LConn1
  ARN-MAN 2*169km/RConn2 -- MAN7/LConn2
  ARN-MAN 2*169km/RConn3 -- MAN7/LConn3
  Cs BER/LConn1 -- 5000 MVA 13.8 kV/735 kV2/RConn1 -- MIC-MAN 60 km/RConn1 -- MAN-MIC 1650 Mvar/LConn1 -- MAN7/RConn1
  Cs BER/LConn2 -- 5000 MVA 13.8 kV/735 kV2/RConn2 -- MIC-MAN 60 km/RConn2 -- MAN-MIC 1650 Mvar/LConn2 -- MAN7/RConn2
  Cs BER/LConn3 -- Load Flow Bus5/LConn1 -- 5000 MVA 13.8 kV/735 kV2/RConn3 -- MIC-MAN 60 km/RConn3 -- MAN-MIC 1650 Mvar/LConn3 -- MAN7/RConn3
  B_7 MAN 5000 MVA/RConn1 -- 5000 MVA 13.8 kV/735 kV2/LConn1 -- 250 MW/LConn1
  B_7 MAN 5000 MVA/RConn2 -- 5000 MVA 13.8 kV/735 kV2/LConn2 -- 250 MW/LConn2
  B_7 MAN 5000 MVA/RConn3 -- 5000 MVA 13.8 kV/735 kV2/LConn3 -- Load Flow Bus3/LConn1 -- 250 MW/LConn3
  MIC-LTD 409 km/RConn2 -- MAN-LEV 3*379km/RConn2 -- QUE7b/RConn1
  Cs ARNS2/LConn1 -- ARN 990 Mvar/LConn1 -- "Cs MTG+ARNN "/RConn1 -- "Cs ARNS1 "/LConn1
  Cs ARNS2/LConn2 -- ARN 990 Mvar/LConn2 -- "Cs MTG+ARNN "/RConn2 -- "Cs ARNS1 "/LConn2
  Cs ARNS2/LConn3 -- Load Flow Bus4/LConn1 -- "Cs ARNS1 "/LConn3 -- ARN 990 Mvar/LConn3 -- "Cs MTG+ARNN "/RConn3
  MIC-LTD 409 km/RConn1 -- QUE7a/RConn1 -- MAN-LEV 3*379km/RConn1
  MIC-LTD 409 km/RConn3 -- QUE7c/RConn1 -- MAN-LEV 3*379km/RConn3
